simulink model "tankdeckel"  (R2015b)
settings: Solver=VariableStepAuto  StartTime=0.0  StopTime=inf  RelTol=1e-3
settings Model: Creator=scco1019  LastModifiedBy=scco1019

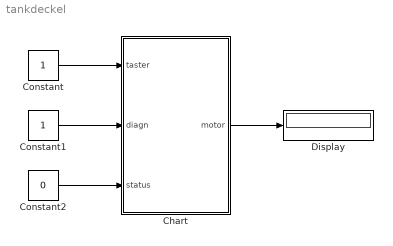
== system tankdeckel ==
  Chart : Stateflow chart  TreatAsAtomicUnit=on
  Constant : Constant
  Constant1 : Constant
  Constant2 : Constant  Value=0
  Display : Display
  wires:
  Chart/1(motor) -> Display/1
  Constant/1 -> Chart/1(taster)
  Constant1/1 -> Chart/2(diagn)
  Constant2/1 -> Chart/3(status)

== stateflow chart tankdeckel/Chart ==
  (default) -> (junction 6)
  (junction 10) -> (junction 18) : {motor = 1}
  (junction 6) -> (junction 10) [order 2] : [status == 0]
  (junction 6) -> (junction 14) [order 3] : {motor = 0}
  (junction 6) -> (junction 8) [order 1] : [(taster==0) || (diagn==0)]
  (junction 8) -> (junction 14) [order 2] : {motor = 0}
  (junction 8) -> (junction 12) [order 1] : [status == 1]
  (junction 12) -> (junction 16) : {motor = 2}
  data: taster input; diagn input; status input; motor output
